simulink model "relayassignment"  (R2019a)
settings: Solver=VariableStepAuto  StartTime=0.0  StopTime=10.0  RelTol=1e-3
libraries: simulink x3
settings Model: Creator=INDIA  LastModifiedBy=INDIA

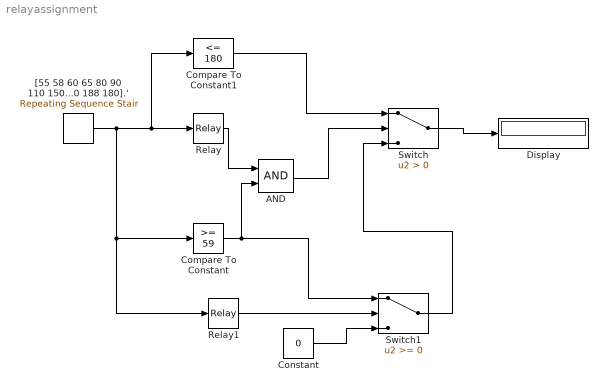
== system relayassignment ==
  AND : Logic  AllPortsSameDT=off  OutDataTypeStr=boolean
  Compare To Constant : simulink/Logic and Bit Operations/Compare To Constant  relop=>=  const=59  OutDataTypeStr=boolean
  Compare To Constant1 : simulink/Logic and Bit Operations/Compare To Constant  relop=<=  const=180  OutDataTypeStr=boolean
  Constant : Constant  Value=0
  Display : Display
  Relay : Relay  OnSwitchValue=60  OffSwitchValue=59
  Relay1 : Relay  OnSwitchValue=181  OffSwitchValue=60  OnOutputValue=0  OffOutputValue=1
  Switch : Switch  Criteria=u2 > Threshold
  Switch1 : Switch
  "[55 58 60 65 80 90 110 150 180 185 190 188 180].'" : simulink/Sources/Repeating Sequence Stair  OutValues=[55 58 60 65 80 90 110 150 180 185 190 188 180].'  tsamp=-1  OutMin=[]  OutMax=[]  OutDataTypeStr=double  OutputDataTypeScalingMode=double  OutDataType=fixdt(0,8)  ConRadixGroup=Best Precision: Vector-wise  OutScaling=2^-12
  wires:
  Switch/1 -> Display/1
  Switch1/1 -> Switch/3
  "[55 58 60 65 80 90 110 150 180 185 190 188 180].'"/1 -> Compare To Constant/1, Relay1/1, Compare To Constant1/1, Relay/1
  Compare To Constant/1 -> Switch1/1, AND/2
  Relay1/1 -> Switch1/2
  Relay/1 -> AND/1
  Constant/1 -> Switch1/3
  AND/1 -> Switch/2
  Compare To Constant1/1 -> Switch/1
